simulink model "FOQL_PDE_StateFeedback"  (R2020a)
settings: Solver=VariableStepAuto  StartTime=0.0  StopTime=10  FixedStep=0.01  MaxStep=0.1  RelTol=1e-5  AbsTol=1e-5
libraries: PDECharactLib x1
settings Model: Creator=kc5492  LastModifiedBy=User
settings SolverCC: ZeroCrossAlgorithm=Adaptive
settings DataIOCC: ReturnWorkspaceOutputs=off
settings DebuggingCC: PregeneratedLibrarySubsystemCodeDiagnostic=none  ArithmeticOperatorsInVariantConditions=warning
settings SFSimCC: SimUseLocalCustomCode=off  CustomCodeUndefinedFunction=UseInterfaceOnly
settings RTWCC: RTWUseLocalCustomCode=off

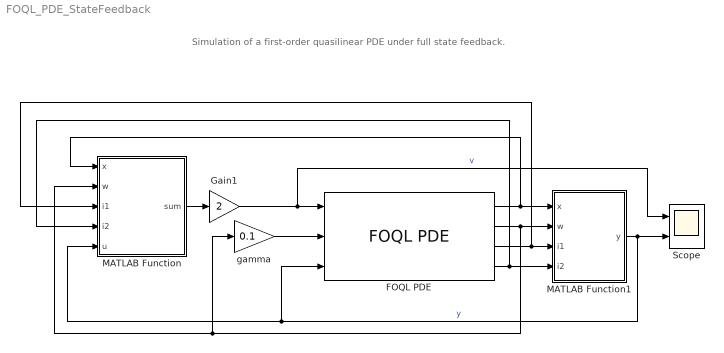
== system FOQL_PDE_StateFeedback ==
  note: Simulation of a first-order quasilinear PDE under full state feedback.
  FOQL PDE : PDECharactLib/FOQL PDE  ell=1  Nmax=100  x0=[0 0.5 0.5 1]  w0=[0 0 1 1]  initX=0  initW=0  dx=0.1  dw=0.01  dt=0.1  crossing_tol=1e-11  overflow_err=off
  Gain1 : Gain  Gain=2
  MATLAB Function : MATLAB Function  TreatAsAtomicUnit=on
  MATLAB Function1 : MATLAB Function  TreatAsAtomicUnit=on
  Scope : Scope  NumInputPorts=2
  gamma : Gain  Gain=0.1
  wires:
  MATLAB Function1/1(y) -> Scope/2, FOQL PDE/3, MATLAB Function/5(u)  "y"
  MATLAB Function/1(sum) -> Gain1/1
  gamma/1 -> FOQL PDE/2
  FOQL PDE/1 -> MATLAB Function1/1(x), MATLAB Function/1(x)
  FOQL PDE/2 -> MATLAB Function1/2(w), MATLAB Function/2(w), gamma/1
  FOQL PDE/3 -> MATLAB Function1/3(i1), MATLAB Function/3(i1)
  Gain1/1 -> FOQL PDE/1, Scope/1  "v"
  FOQL PDE/4 -> MATLAB Function1/4(i2), MATLAB Function/4(i2)

== matlab function FOQL_PDE_StateFeedback/MATLAB Function ==
  data: x input; sum output; w input; i1 input; i2 input; u input
function sum = integral(x, w, i1, i2, u)

if i1 < i2
    ind = i1:i2;
else
    ind = [i1:length(x), 1:i2];
end

w = [u; w(ind(1:end-1)); interp1(x(ind) + 1e-11*(0:length(ind)-1)', w(ind), 1)];
x = [0; x(ind(1:end-1)); 1];

sum = trapz(x, w);

== matlab function FOQL_PDE_StateFeedback/MATLAB Function1 ==
  data: x input; y output; w input; i1 input; i2 input
function y = output(x, w, i1, i2)

if i1 < i2
    ind = i1:i2;
else
    ind = [i1:length(x), 1:i2];
end

y = interp1(x(ind) + 1e-11*(0:length(ind)-1)', w(ind), 1);
